simulink model "fiber1"  (R2017b)
settings: Solver=FixedStepAuto  StartTime=-40  StopTime=39.921875  FixedStep=0.078125  RelTol=1e-3
undefined symbols (not defined in the file or in its folder): magnitude
libraries: dspxfrm3 x4
settings Model: Creator=June  LastModifiedBy=njc
settings SolverCC: DecoupledContinuousIntegration=on
settings OptimizationCC: DefaultParameterBehavior=Inlined  UseDivisionForNetSlopeComputation=on  UseFloatMulNetSlope=on  InlineInvariantSignals=on  PassReuseOutputArgsAs=Individual arguments  ZeroExternalMemoryAtStartup=off  ZeroInternalMemoryAtStartup=off  NoFixptDivByZeroProtection=on  EfficientFloat2IntCast=on  LifeSpan=1
settings DebuggingCC: AlgebraicLoopMsg=none  ArtificialAlgebraicLoopMsg=none  MaxConsecutiveZCsMsg=none  ParameterTunabilityLossMsg=error  ModelReferenceExtraNoncontSigs=none  SimStateInterfaceChecksumMismatchMsg=none  ForceCombineOutputUpdateInSim=on
settings HardwareCC: ProdLongLongMode=on
settings SFSimCC: MATLABDynamicMemAlloc=off
settings RTWCC: SystemTargetFile=ert.tlc  TemplateMakefile=ert_default_tmf  GenerateReport=on  IncludeHyperlinkInReport=on  LaunchReport=on  GenerateTraceInfo=on  GenerateTraceReport=on  GenerateTraceReportSl=on  GenerateTraceReportSf=on  GenerateTraceReportEml=on  GenerateCodeMetricsReport=on
settings CodeAppCC: ForceParamTrailComments=on  IgnoreCustomStorageClasses=off  OperatorAnnotations=on  SimulinkDataObjDesc=on  SFDataObjDesc=on  CustomSymbolStrGlobalVar=rt$N$M  CustomSymbolStrType=$N$M  CustomSymbolStrFcn=$N$M$F  CustomSymbolStrMacro=$N$M  InsertBlockDesc=on
settings ERTTargetCC: TargetLangStandard=C99 (ISO)  GenerateSampleERTMain=on  IncludeMdlTerminateFcn=off  CombineSignalStateStructs=on  SupportContinuousTime=on  SupportNonInlinedSFcns=on  InlinedParameterPlacement=NonHierarchical  ERTCustomFileTemplate=example_file_process.tlc  ERTFilePackagingFormat=CompactWithDataFile

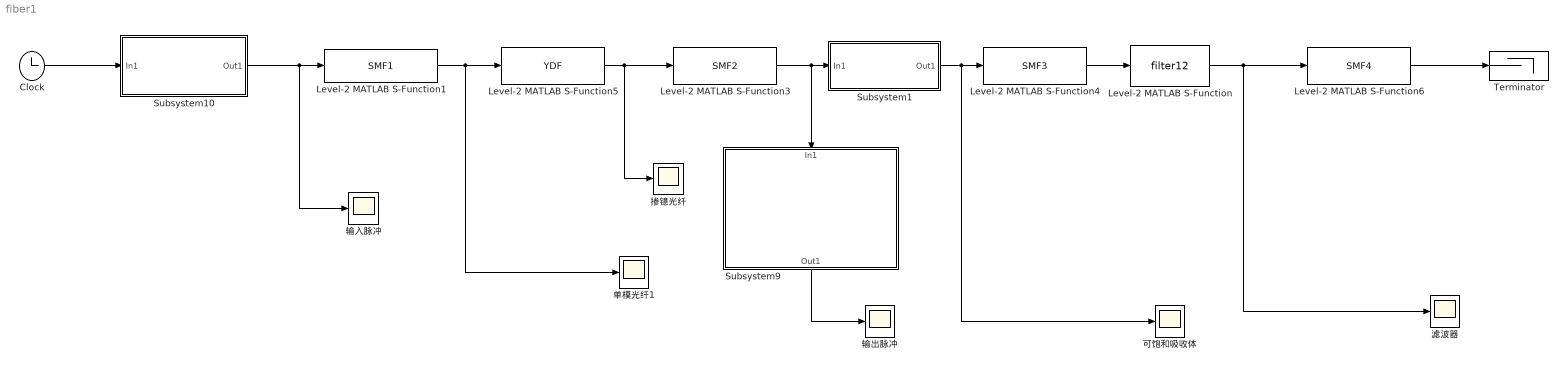
== system fiber1 ==
  Clock : Clock
      settings: Decimation=1024
  Level-2 MATLAB S-Function : M-S-Function  FunctionName=filter12
  Level-2 MATLAB S-Function1 : M-S-Function  FunctionName=SMF1
  Level-2 MATLAB S-Function3 : M-S-Function  FunctionName=SMF2
  Level-2 MATLAB S-Function4 : M-S-Function  FunctionName=SMF3
  Level-2 MATLAB S-Function5 : M-S-Function  FunctionName=YDF
  Level-2 MATLAB S-Function6 : M-S-Function  FunctionName=SMF4
  Subsystem1 : Subsystem  mask{g_Md=0.05, g_Ps=20, g_A_ns=0.4, g_cc=0.8}
      mask prompts: g_Md "Md"; g_Ps "Ps"; g_A_ns "A_ns"; g_cc "cc"
      mask Display: disp('absorber')
  Subsystem10 : Subsystem
      mask Display: disp('输入脉冲')
  Subsystem9 : Subsystem  mask{g_cc=0.8}
      mask prompts: g_cc "cc"
      mask Display: disp('Output Coupler')
  Terminator : Terminator
  单模光纤1 : Scope
  可饱和吸收体 : Scope
  掺镱光纤 : Scope
  滤波器 : Scope
  输入脉冲 : Scope
  输出脉冲 : Scope
  wires:
  Subsystem1/1(Out1) -> 可饱和吸收体/1, Level-2 MATLAB S-Function4/1
  Level-2 MATLAB S-Function1/1 -> Level-2 MATLAB S-Function5/1, 单模光纤1/1
  Level-2 MATLAB S-Function3/1 -> Subsystem9/1(In1), Subsystem1/1(In1)
  Subsystem10/1(Out1) -> 输入脉冲/1, Level-2 MATLAB S-Function1/1
  Clock/1 -> Subsystem10/1(In1)
  Level-2 MATLAB S-Function4/1 -> Level-2 MATLAB S-Function/1
  Level-2 MATLAB S-Function6/1 -> Terminator/1
  Level-2 MATLAB S-Function/1 -> 滤波器/1, Level-2 MATLAB S-Function6/1
  Level-2 MATLAB S-Function5/1 -> 掺镱光纤/1, Level-2 MATLAB S-Function3/1
  Subsystem9/1(Out1) -> 输出脉冲/1

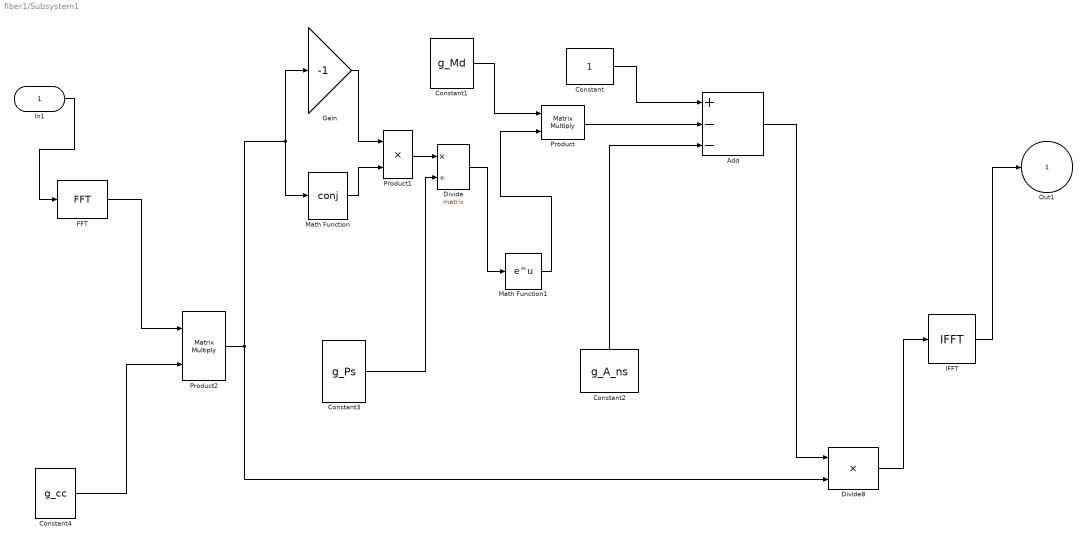
== system fiber1/Subsystem1 ==
  In1 : Inport
  Add : Sum  Inputs=+--
  Constant : Constant
  Constant1 : Constant  Value=g_Md
  Constant2 : Constant  Value=g_A_ns
  Constant3 : Constant  Value=g_Ps
  Constant4 : Constant  Value=g_cc
  Divide : Product  Inputs=*/  Multiplication=Matrix(*)
  Divide8 : Product  Inputs=**
  FFT : dspxfrm3/FFT  FFTImplementation=Auto  CompMethod=Table lookup  TableOpt=NEW  TableOptActive=Speed  BitRevOrder=off  Normalize=off  InheritFFTLength=on  FFTLength=64  WrapInput=on  roundingMode=Floor  overflowMode=off  firstCoeffDataTypeStr=Inherit: Same word length as input  firstCoeffLastDataTypeStr=Inherit: Same word length as input  outputMin=[]  outputMax=[]
  Gain : Gain  Gain=-1
  IFFT : dspxfrm3/IFFT  FFTImplementation=Auto  CompMethod=Table lookup  TableOpt=NEW  TableOptActive=Speed  BitRevOrder=off  cs_in=off  Normalize=on  InheritFFTLength=on  FFTLength=64  WrapInput=on  mode=Complex  outSamplingMode=Sample based  roundingMode=Floor  overflowMode=off  firstCoeffDataTypeStr=Inherit: Same word length as input  firstCoeffLastDataTypeStr=Inherit: Same word length as input  outputMin=[]  outputMax=[]
      settings: SourceProductName=DSP System Toolbox
  Math Function : Math  Operator=conj  SaturateOnIntegerOverflow=on
  Math Function1 : Math  SaturateOnIntegerOverflow=on
  Product : Product  Multiplication=Matrix(*)
  Product1 : Product
  Product2 : Product  Multiplication=Matrix(*)
  Out1 : Outport
  wires:
  Constant1/1 -> Product/1
  Math Function1/1 -> Product/2
  Product1/1 -> Divide/1
  Constant3/1 -> Divide/2
  Constant/1 -> Add/1
  Gain/1 -> Product1/1
  Math Function/1 -> Product1/2
  Divide/1 -> Math Function1/1
  Constant2/1 -> Add/3
  Product/1 -> Add/2
  Add/1 -> Divide8/1
  Product2/1 -> Math Function/1, Gain/1, Divide8/2
  Constant4/1 -> Product2/2
  In1/1 -> FFT/1
  FFT/1 -> Product2/1
  Divide8/1 -> IFFT/1
  IFFT/1 -> Out1/1

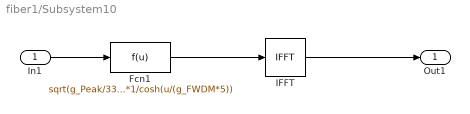
== system fiber1/Subsystem10 ==
  In1 : Inport
  Fcn1 : Fcn  Expr=sqrt(g_Peak/339)*1/cosh(u/(g_FWDM*5))  mask{g_Peak=100, g_FWDM=2}
      mask prompts: g_Peak "Peak"; g_FWDM "FWDM"
      mask Display: disp('sech')
  IFFT : dspxfrm3/IFFT  FFTImplementation=Auto  CompMethod=Table lookup  TableOpt=NEW  TableOptActive=Speed  BitRevOrder=off  cs_in=off  Normalize=on  InheritFFTLength=on  FFTLength=64  WrapInput=on  mode=Complex  outSamplingMode=Sample based  roundingMode=Floor  overflowMode=off  firstCoeffDataTypeStr=Inherit: Same word length as input  firstCoeffLastDataTypeStr=Inherit: Same word length as input  outputMin=[]  outputMax=[]
      settings: SourceProductName=DSP System Toolbox
  Out1 : Outport
  wires:
  In1/1 -> Fcn1/1
  Fcn1/1 -> IFFT/1
  IFFT/1 -> Out1/1

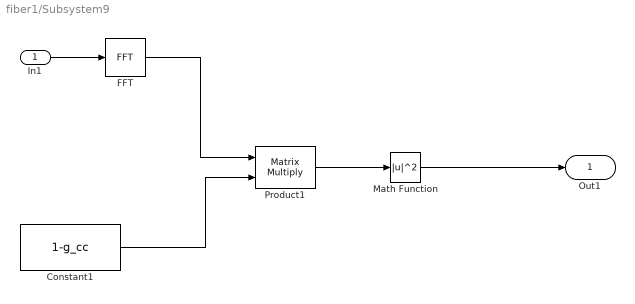
== system fiber1/Subsystem9 ==
  In1 : Inport
  Constant1 : Constant  Value=1-g_cc
  FFT : dspxfrm3/FFT  FFTImplementation=Auto  CompMethod=Table lookup  TableOpt=NEW  TableOptActive=Speed  BitRevOrder=off  Normalize=off  InheritFFTLength=on  FFTLength=64  WrapInput=on  roundingMode=Floor  overflowMode=off  firstCoeffDataTypeStr=Inherit: Same word length as input  firstCoeffLastDataTypeStr=Inherit: Same word length as input  outputMin=[]  outputMax=[]
  Math Function : Math  Operator=magnitude^2  SaturateOnIntegerOverflow=on
  Product1 : Product  Multiplication=Matrix(*)
  Out1 : Outport
  wires:
  Constant1/1 -> Product1/2
  Product1/1 -> Math Function/1
  Math Function/1 -> Out1/1
  In1/1 -> FFT/1
  FFT/1 -> Product1/1
